simulink model "lookup_nD_TestGen37"  (R2017b)
settings: Solver=FixedStepDiscrete  StartTime=0.0  StopTime=10.0  RelTol=1e-3
settings Model: Creator=ktrinh  LastModifiedBy=ktrinh
settings DebuggingCC: ParameterOverflowMsg=none

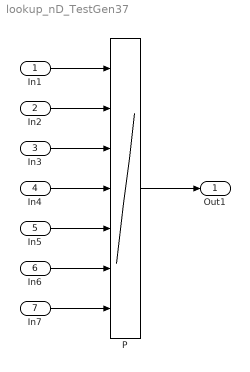
== system lookup_nD_TestGen37 ==
  In1 : Inport  OutMin=0  OutMax=127  OutDataTypeStr=uint8  PortDimensions=1
  In2 : Inport  Port=2  OutMin=0  OutMax=127  OutDataTypeStr=uint8
  In3 : Inport  Port=3  OutMin=0  OutMax=127  OutDataTypeStr=uint8
  In4 : Inport  Port=4  OutMin=0  OutMax=127  OutDataTypeStr=uint8
  In5 : Inport  Port=5  OutMin=0  OutMax=127  OutDataTypeStr=uint8
  In6 : Inport  Port=6  OutMin=0  OutMax=127  OutDataTypeStr=uint8
  In7 : Inport  Port=7  OutMin=0  OutMax=127  OutDataTypeStr=uint8
  P : Lookup_n-D  NumberOfTableDimensions=7  BreakpointsForDimension1=[63.9654193163996;73.0578880846683]  BreakpointsForDimension2=[15.7308247792324;65.1500336115267;69.9525901439905;96.166286485537;103.346190842451]  BreakpointsForDimension3=[4.34102484866711;23.4195110124267;36.471437864466]  BreakpointsForDimension4=[40.8032410554062;57.8366289718747]  BreakpointsForDimension5=[5.86615162815535;46.4557959549338;53.0735865108056]  BreakpointsForDimension6=[31.8007410978587;37.4328396737041;56.968506493087;89.9665888221587]  BreakpointsForDimension7=[9.57919393811142;42.6630668457541;49.4350203254805]  BreakpointsForDimension1DataTypeStr=uint16  BreakpointsForDimension2DataTypeStr=uint16  BreakpointsForDimension3DataTypeStr=uint16  BreakpointsForDimension4DataTypeStr=uint16  BreakpointsForDimension5DataTypeStr=uint16  BreakpointsForDimension6DataTypeStr=uint16  BreakpointsForDimension7DataTypeStr=uint16  Table=reshape(repmat([4 5 6 7 8;16 19 20 21 22;10 18 23 24 25],18,8),[2,5,3,2,3,4,3])  TableDataTypeStr=single  InterpMethod=Flat  ExtrapMethod=Clip  InternalRulePriority=Speed  OutDataTypeStr=uint16  SaturateOnIntegerOverflow=on  InputSameDT=on
  Out1 : Outport
  wires:
  In1/1 -> P/1
  In2/1 -> P/2
  In3/1 -> P/3
  In4/1 -> P/4
  In5/1 -> P/5
  In6/1 -> P/6
  In7/1 -> P/7
  P/1 -> Out1/1
